simulink model "MS_SPI_Protocol"  (R2021b)
settings: Solver=VariableStepAuto  StartTime=0.0  StopTime=10.0  RelTol=1e-3
settings Model: Creator=CPcom  LastModifiedBy=CPcom

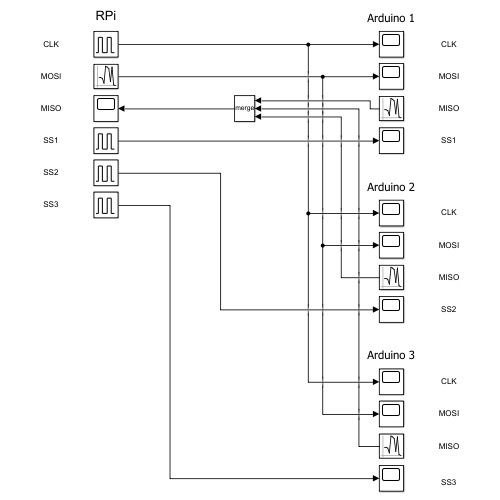
[thumbnail: Simulink's stored preview of the top-level diagram]
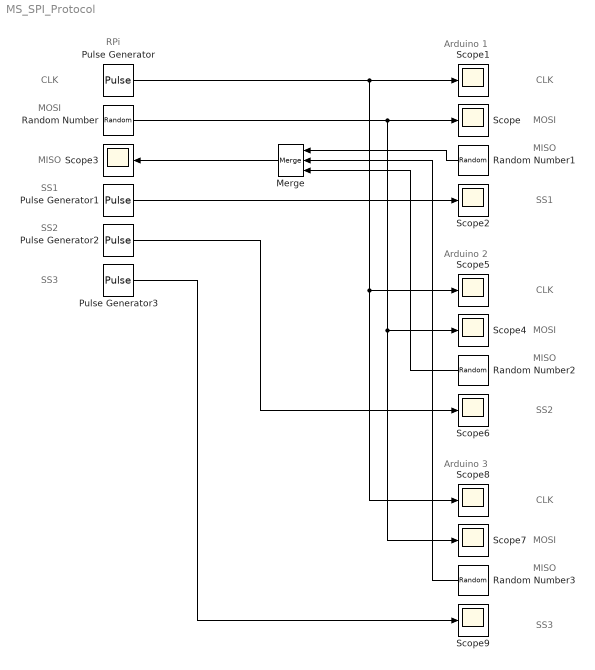
== system MS_SPI_Protocol ==
  note: Arduino 1
  note: RPi
  note: SS2
  note: SS1
  note: MISO
  note: MOSI
  note: CLK
  note: SS3
  note: MISO
  note: MOSI
  note: CLK
  note: MISO
  note: MOSI
  note: CLK
  note: MISO
  note: MOSI
  note: CLK
  note: SS1
  note: SS2
  note: SS3
  note: Arduino 2
  note: Arduino 3
  Merge : Merge  Inputs=3
  Pulse Generator{,1..3} (4 alike) : DiscretePulseGenerator  PulseType=Time based  Period=10  PulseWidth=5
  Random Number{,1..3} (4 alike) : RandomNumber  SampleTime=0.1
  Scope{,1..9} (10 alike) : Scope
  wires:
  Random Number/1 -> Scope/1, Scope7/1, Scope4/1
  Pulse Generator1/1 -> Scope2/1
  Random Number1/1 -> Merge/1
  Random Number3/1 -> Merge/2
  Random Number2/1 -> Merge/3
  Merge/1 -> Scope3/1
  Pulse Generator2/1 -> Scope6/1
  Pulse Generator3/1 -> Scope9/1
  Pulse Generator/1 -> Scope8/1, Scope5/1, Scope1/1
